simulink model "pendcart_2016"  (Simulink 8.8)
settings: Solver=ode45  StartTime=0.0  StopTime=tsim  RelTol=1e-3  EnableMultiTasking=on
values from neighbouring files (symbols this model uses):
  b = 0.01    [pendcartsim.m]
  c = 0.05    [pendcartsim.m]
  g = 9.82    [pendcartsim.m]
  K1 = -119.0071    [pendcartsim.m]
  K2 = 0.0402    [pendcartsim.m]
  l = 0.5    [pendcartsim.m]
  M = 1.2    [pendcartsim.m]
  m = 0.2    [pendcartsim.m]
  p = 5.4277    [pendcartsim.m]
  p1 = 25.4277    [pendcartsim.m]
  theta0 = 5*pi/180    (= 0.0872664625997)    [pendcartsim.m]
settings Model: SuppressorTable=22 serialization::archive 11 0 6 0 0 0 8 0  Creator=Chris  LastModifiedBy=Administrator
settings OptimizationCC: ExpressionDepthLimit=2147483647  InitFltsAndDblsToZero=on
settings DebuggingCC: AlgebraicLoopMsg=none  SaveWithParameterizedLinksMsg=none
settings GRTTargetCC: TargetFcnLib=ansi_tfl_tmw.mat

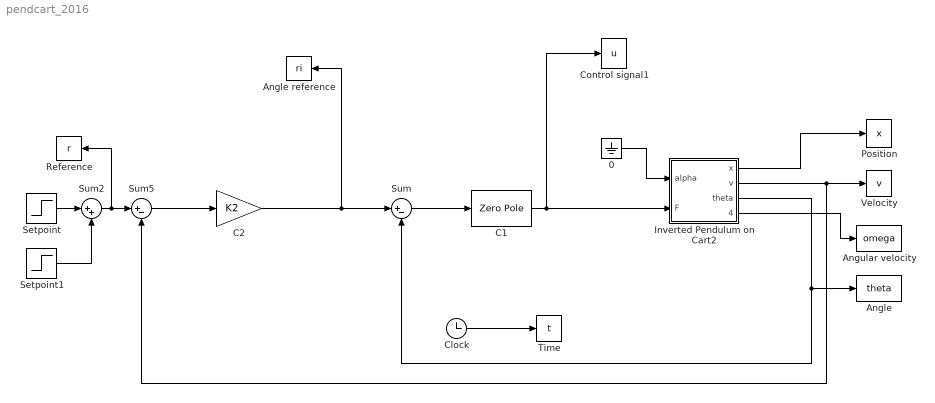
== system pendcart_2016 ==
  0 : Ground
  Angle : ToWorkspace  VariableName=theta  SampleTime=-1
  Angle reference : ToWorkspace  VariableName=ri  SampleTime=-1
  Angular velocity : ToWorkspace  VariableName=omega  SampleTime=-1
  C1 : ZeroPole  Zeros=[-p]  Poles=[-p1]  Gain=[K1]
  C2 : Gain  Gain=K2
  Clock : Clock
  Control signal1 : ToWorkspace  VariableName=u  SampleTime=-1
  Inverted Pendulum on Cart2 : Subsystem
  Position : ToWorkspace  VariableName=x  SampleTime=-1
  Reference : ToWorkspace  VariableName=r  SampleTime=-1
  Setpoint : Step  Time=10  After=0.5  SampleTime=0
  Setpoint1 : Step  Time=20  After=-0.5  SampleTime=0
  Sum : Sum  Inputs=|+-
  Sum2 : Sum  Inputs=|++
  Sum5 : Sum  Inputs=|+-
  Time : ToWorkspace  VariableName=t  SampleTime=-1
  Velocity : ToWorkspace  VariableName=v  SampleTime=-1
  wires:
  Clock/1 -> Time/1
  Inverted Pendulum on Cart2/1(x) -> Position/1
  Sum/1 -> C1/1
  C1/1 -> Inverted Pendulum on Cart2/2(F), Control signal1/1
  Inverted Pendulum on Cart2/4(omega) -> Angular velocity/1
  Inverted Pendulum on Cart2/2(v) -> Velocity/1, Sum5/2
  Inverted Pendulum on Cart2/3(theta) -> Angle/1, Sum/2
  Sum5/1 -> C2/1
  C2/1 -> Angle reference/1, Sum/1
  Setpoint/1 -> Sum2/1
  Setpoint1/1 -> Sum2/2
  Sum2/1 -> Sum5/1, Reference/1
  0/1 -> Inverted Pendulum on Cart2/1(alpha)

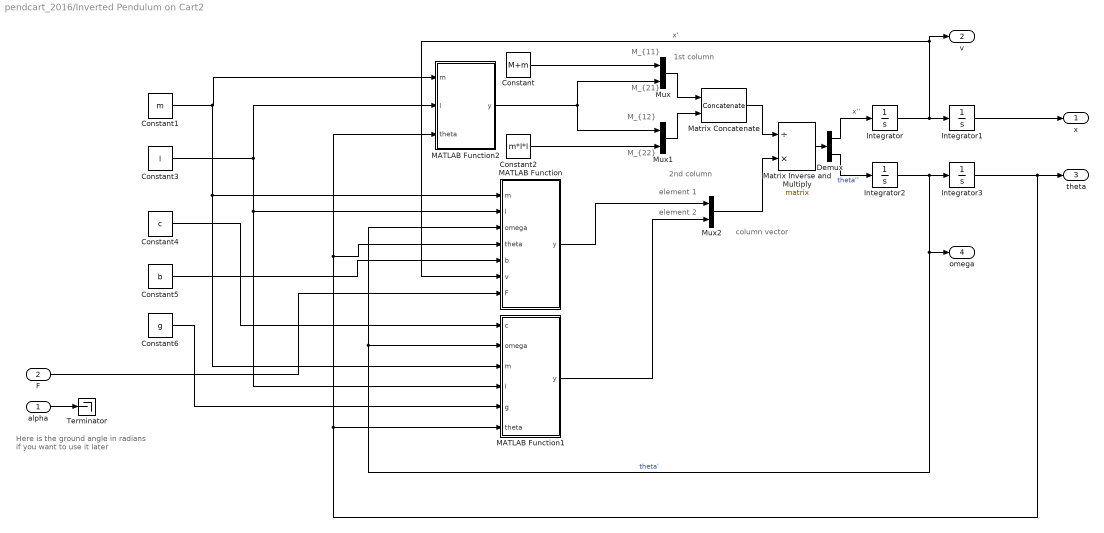
== system pendcart_2016/Inverted Pendulum on Cart2 ==
  note: 2nd column
  note: M_{21}
  note: 1st column
  note: M_{12}
  note: element 2
  note: Here is the ground angle in
      | radians if you want to use it later
  note: column vector
  note: M_{11}
  note: M_{22}
  note: element 1
  alpha : Inport
  F : Inport  Port=2
  Constant : Constant  Value=M+m
  Constant1 : Constant  Value=m
  Constant2 : Constant  Value=m*l*l
  Constant3 : Constant  Value=l
  Constant4 : Constant  Value=c
  Constant5 : Constant  Value=b
  Constant6 : Constant  Value=g
  Demux : Demux  Outputs=2
  Integrator : Integrator
  Integrator1 : Integrator
  Integrator2 : Integrator
  Integrator3 : Integrator  InitialCondition=theta0
  MATLAB Function : MATLAB Function  TreatAsAtomicUnit=on
  MATLAB Function1 : MATLAB Function  TreatAsAtomicUnit=on
  MATLAB Function2 : MATLAB Function  TreatAsAtomicUnit=on
  Matrix Concatenate : Concatenate  Mode=Multidimensional array  ConcatenateDimension=2
  Matrix Inverse and Multiply : Product  Inputs=/*  Multiplication=Matrix(*)
  Mux : Mux  Inputs=2
  Mux1 : Mux  Inputs=2
  Mux2 : Mux  Inputs=2
  Terminator : Terminator
  x : Outport
  v : Outport  Port=2
  theta : Outport  Port=3
  omega : Outport  Port=4
  wires:
  F/1 -> MATLAB Function/7(F)
  MATLAB Function1/1(y) -> Mux2/2
  Constant1/1 -> MATLAB Function1/3(m), MATLAB Function/1(m), MATLAB Function2/1(m)
  Constant5/1 -> MATLAB Function/5(b)
  Matrix Inverse and Multiply/1 -> Demux/1
  Constant2/1 -> Mux1/2
  Mux2/1 -> Matrix Inverse and Multiply/2
  MATLAB Function/1(y) -> Mux2/1
  Constant4/1 -> MATLAB Function1/1(c)
  Mux1/1 -> Matrix Concatenate/2
  Constant/1 -> Mux/1
  MATLAB Function2/1(y) -> Mux1/1, Mux/2
  Integrator/1 -> Integrator1/1, v/1, MATLAB Function/6(v)  "x'"
  Matrix Concatenate/1 -> Matrix Inverse and Multiply/1
  Integrator1/1 -> x/1
  Demux/2 -> Integrator2/1  "theta''"
  Integrator3/1 -> MATLAB Function/4(theta), MATLAB Function2/3(theta), MATLAB Function1/6(theta), theta/1
  Constant3/1 -> MATLAB Function1/4(l), MATLAB Function/2(l), MATLAB Function2/2(l)
  Mux/1 -> Matrix Concatenate/1
  Integrator2/1 -> Integrator3/1, MATLAB Function/3(omega), MATLAB Function1/2(omega), omega/1  "theta'"
  Constant6/1 -> MATLAB Function1/5(g)
  alpha/1 -> Terminator/1
  Demux/1 -> Integrator/1  "x''"

== matlab function Inverted Pendulum on Cart2/MATLAB Function1 ==
  data: y output double; c input double; omega input double; m input double; l input double; g input double; theta input double
function y  = fcn(c,omega,m,l,g,theta)

y =c*omega+m*l*g*sin(theta);

== matlab function Inverted Pendulum on Cart2/MATLAB Function ==
  data: y output double; m input double; l input double; omega input double; theta input double; b input double; v input double; F input double
function y = fcn(m,l,omega,theta,b,v,F)

y =m*l*omega*omega*sin(theta)+b*v+F;

== matlab function Inverted Pendulum on Cart2/MATLAB Function2 ==
  data: y output double; m input double; l input double; theta input double
function y = fcn(m,l,theta)

y =m*l*cos(theta);
